simulink library "common_lib"  (R2021b)
settings: Solver=ode45  StartTime=0.0  StopTime=10.0  RelTol=1e-3
undefined symbols (not defined in the file or in its folder): ACCEL_PRE_MULT, C_C1GearNumbers, C_C1GearRatios, C_Calibration, C_DitherWaveform, C_GearOffset, C_GearRatioIn, C_GearRatioInverseOut, C_GearRatioOut, CLUTCH_INNER_LOOP_UPDATE_RATE, CONSTANT, DEGRADED_MODE_SIZE, Dem_EventStatusType, DiscIntNeverNeededParam, F_FAULT_ENUM, F_NOFAULT, F_OUTOFRANGE, F_RATELIMIT, FALSE, FMI14_SPECIAL_INSTRUCTIONS, FMI20_DATA_DRIFTED_HIGH, FMI21_DATA_DRIFTED_LOW, FMI29_RESERVED_FOR_SAE_ASSIGNMENT, FMI30_RESERVED_FOR_SAE_ASSIGNMENT, FMI31_CONDITION_EXISTS, FMI32_NO_FAULT, IC, k_accel, k_mean, LVDCU_OORH_FaultCntThd_C, MAX_UINT32, MEAN_PRE_MULT, NTriggers, QLTY_SIGNAL_FAILED, QLTY_SIGNAL_FULLY_FUNCTION, QLTY_SIGNAL_SUBSTITUTED_BY_1ST_CHOICE, QLTY_SIGNAL_SUBSTITUTED_BY_2ND_CHOICE, QLTY_SIGNAL_SUBSTITUTED_BY_3RD_CHOICE, QLTY_SIGNAL_SUBSTITUTED_BY_4TH_CHOICE, SAMPLE_TIME_100_mSec, SAMPLE_TIME_100_uSec, simin, T_TestPoint, TF_FALSE, TF_TRUE, TimeStep, TRUE, WORKSPACE_UPDATE_RATE, ZERO, Zero
libraries: $bdroot x120, simulink x27, simulink_extras x4, MBD_EPS_Local_Blockset x4
(part 10 of 10)

== stateflow chart common_lib/Diagnostics/DiagcFltStSpaceHoldCnt/diagcounter_hold ==
  state Init
    en: diagFaultCnt = int16(0);
    diagFaultStatus = PASSED;
    Init -> (junction 169) [order 1]
    (junction 169) -> (junction 170) [order 1] : [~diagStartUpComp || diagReset]
        | {diagFaultCnt = int16(0);}
    (junction 169) -> (junction 171) [order 2]
    (junction 170) -> (junction 180)
    (junction 171) -> (junction 172) [order 1] : [~diagFaultActive]
    (junction 171) -> (junction 173) [order 2]
    (junction 172) -> (junction 179) : {diagFaultCnt = diagFaultCnt;}
    (junction 173) -> (junction 174) [order 1] : [diagFaultActive]
    (junction 174) -> (junction 175) [order 1] : [diagFaultCnt>=diagFaultCntThresh]
        | {diagFaultStatus = FAILED}
    (junction 173) -> (junction 176) [order 2]
    (junction 174) -> (junction 177) [order 2] : {diagFaultCnt = diagFaultCnt + diagUpCnt;}
    (junction 175) -> (junction 178)
    (junction 177) -> (junction 176)
    (junction 178) -> (junction 177)
    (junction 179) -> (junction 178)
    (junction 180) -> (junction 179)
    (junction 176) -> (junction 181)
  state Fault
    en:
    diagFaultStatus = FAILED ;
    Fault -> (junction 200) [order 1]
    (junction 200) -> (junction 201) [order 1] : [(diagFaultCnt<diagFaultCntThresh) && diagFaultActive]
        | {diagFaultCnt = diagFaultCnt + diagUpCnt;}
    (junction 200) -> (junction 202) [order 2]
    (junction 201) -> (junction 203)
    (junction 203) -> (junction 202)
    (junction 202) -> (junction 204)
  state Pass
    en: diagFaultCnt = int16(0);
    diagFaultStatus = PASSED;
    Pass -> (junction 212) [order 1]
    (junction 212) -> (junction 213) [order 1] : [(diagFaultCnt>int16(0)) && ~diagFaultActive]
        | {diagFaultCnt = diagFaultCnt;}
    (junction 212) -> (junction 215) [order 2]
    (junction 213) -> (junction 221)
    (junction 215) -> (junction 216) [order 1] : [diagFaultActive]
    (junction 216) -> (junction 217) [order 1] : [diagFaultCnt>=diagFaultCntThresh]
        | {diagFaultStatus = FAILED;}
    (junction 215) -> (junction 218) [order 2]
    (junction 216) -> (junction 219) [order 2] : {diagFaultCnt = diagFaultCnt + diagUpCnt;}
    (junction 217) -> (junction 220)
    (junction 219) -> (junction 218)
    (junction 220) -> (junction 219)
    (junction 221) -> (junction 220)
    (junction 218) -> (junction 223)
  (default) -> Init : {diagFaultStatus = PASSED
      | diagFaultCnt = int16(0)}
  Init -> Fault [order 1] : [diagFaultCnt>=diagFaultCntThresh &&...
      | diagStartUpComp &&...
      | ~diagReset]
  Fault -> Init [order 2] : [~diagStartUpComp ||...
      | diagReset]
  Fault -> Pass [order 1] : [diagReset]
  Pass -> Fault [order 1] : [diagFaultCnt>=diagFaultCntThresh]
  Init -> Pass [order 2] : [diagFaultCnt==0&&...
      | diagStartUpComp...
      |  &&~diagReset]
  Pass -> Init [order 2] : [~diagStartUpComp ||...
      | diagReset]
  data: diagFaultActive input; diagStartUpComp input; diagUpCnt input; diagFaultCntThresh input; diagReset input; diagFaultStatus output; diagFaultCnt output; FAILED constant boolean =1; PASSED constant boolean =0

== stateflow chart common_lib/Bit/uint8 Bit Pack ==
  settings: stateMachineType=MEALY_MACHINE
  (default) -> (junction 10) : {Byte=0;}
  (junction 10) -> (junction 13) [order 1] : [Bit_0]{Byte=Byte | 1;}
  (junction 10) -> (junction 13) [order 2]
  (junction 13) -> (junction 20) [order 1] : [Bit_1]{Byte=Byte | 2;}
  (junction 13) -> (junction 20) [order 2]
  (junction 20) -> (junction 26) [order 1] : [Bit_2]{Byte=Byte | 4;}
  (junction 20) -> (junction 26) [order 2]
  (junction 26) -> (junction 31) [order 1] : [Bit_3]{Byte=Byte | 8;}
  (junction 26) -> (junction 31) [order 2]
  (junction 31) -> (junction 36) [order 1] : [Bit_4]{Byte=Byte | 16;}
  (junction 31) -> (junction 36) [order 2]
  (junction 36) -> (junction 41) [order 1] : [Bit_5]{Byte=Byte | 32;}
  (junction 36) -> (junction 41) [order 2]
  (junction 41) -> (junction 46) [order 1] : [Bit_6]{Byte=Byte | 64;}
  (junction 41) -> (junction 46) [order 2]
  (junction 46) -> (junction 51) [order 1] : [Bit_7]{Byte=Byte | 128;}
  (junction 46) -> (junction 51) [order 2]
  data: Bit_0 input boolean size=1; Bit_1 input boolean size=1; Bit_2 input boolean size=1; Bit_3 input boolean size=1; Bit_4 input boolean size=1; Bit_5 input boolean size=1; Bit_6 input boolean size=1; Bit_7 input boolean size=1; Byte output uint8 size=1

== stateflow chart common_lib/Bit/uint8 Bit Unpack ==
  settings: stateMachineType=MEALY_MACHINE
  (default) -> (junction 17) : {Bit_0 = Byte & 1;
      |  Bit_1 = Byte & 2;
      |  Bit_2 = Byte & 4;
      |  Bit_3 = Byte & 8;
      |  Bit_4 = Byte & 16;
      |  Bit_5 = Byte & 32;
      |  Bit_6 = Byte & 64;
      |  Bit_7 = Byte & 128;}
  data: Byte input uint8 size=1; Bit_0 output boolean size=1; Bit_1 output boolean size=1; Bit_2 output boolean size=1; Bit_3 output boolean size=1; Bit_4 output boolean size=1; Bit_5 output boolean size=1; Bit_6 output boolean size=1; Bit_7 output boolean size=1

== stateflow chart common_lib/Bit/uint16 Bit Pack ==
  settings: stateMachineType=MEALY_MACHINE
  (default) -> (junction 10) : {Byte=0;}
  (junction 10) -> (junction 13) [order 1] : [Bit_0]{Byte=Byte | 1;}
  (junction 10) -> (junction 13) [order 2]
  (junction 13) -> (junction 20) [order 1] : [Bit_1]{Byte=Byte | 2;}
  (junction 13) -> (junction 20) [order 2]
  (junction 20) -> (junction 26) [order 1] : [Bit_2]{Byte=Byte | 4;}
  (junction 20) -> (junction 26) [order 2]
  (junction 26) -> (junction 31) [order 1] : [Bit_3]{Byte=Byte | 8;}
  (junction 26) -> (junction 31) [order 2]
  (junction 31) -> (junction 36) [order 1] : [Bit_4]{Byte=Byte | 16;}
  (junction 31) -> (junction 36) [order 2]
  (junction 36) -> (junction 41) [order 1] : [Bit_5]{Byte=Byte | 32;}
  (junction 36) -> (junction 41) [order 2]
  (junction 41) -> (junction 46) [order 1] : [Bit_6]{Byte=Byte | 64;}
  (junction 41) -> (junction 46) [order 2]
  (junction 46) -> (junction 65) [order 1] : [Bit_7]{Byte=Byte | 128;}
  (junction 46) -> (junction 65) [order 2]
  (junction 65) -> (junction 66) [order 1] : [Bit_8]{Byte=Byte | 256;}
  (junction 65) -> (junction 66) [order 2]
  (junction 66) -> (junction 69) [order 1] : [Bit_9]{Byte=Byte | 512;}
  (junction 66) -> (junction 69) [order 2]
  (junction 69) -> (junction 72) [order 1] : [Bit_10]{Byte=Byte | 1024;}
  (junction 69) -> (junction 72) [order 2]
  (junction 72) -> (junction 73) [order 1] : [Bit_11]{Byte=Byte | 2048;}
  (junction 72) -> (junction 73) [order 2]
  (junction 73) -> (junction 68) [order 1] : [Bit_12]{Byte=Byte | 4096;}
  (junction 73) -> (junction 68) [order 2]
  (junction 68) -> (junction 71) [order 1] : [Bit_13]{Byte=Byte | 8192;}
  (junction 68) -> (junction 71) [order 2]
  (junction 71) -> (junction 70) [order 1] : [Bit_14]{Byte=Byte | 16384;}
  (junction 71) -> (junction 70) [order 2]
  (junction 70) -> (junction 67) [order 1] : [Bit_15]{Byte=Byte | 32768;}
  (junction 70) -> (junction 67) [order 2]
  data: Bit_0 input boolean size=1; Bit_1 input boolean size=1; Bit_2 input boolean size=1; Bit_3 input boolean size=1; Bit_4 input boolean size=1; Bit_5 input boolean size=1; Bit_6 input boolean size=1; Bit_7 input boolean size=1; Byte output uint16 size=1; Bit_8 input boolean size=1; Bit_9 input boolean size=1; Bit_10 input boolean size=1; Bit_11 input boolean size=1; Bit_12 input boolean size=1; Bit_13 input boolean size=1; Bit_14 input boolean size=1; Bit_15 input boolean size=1

== stateflow chart common_lib/Bit/uint16 Bit Unpack ==
  settings: stateMachineType=MEALY_MACHINE
  (default) -> (junction 17) : {Bit_0 = Byte & 1;
      |  Bit_1 = Byte & 2;
      |  Bit_2 = Byte & 4;
      |  Bit_3 = Byte & 8;
      |  Bit_4 = Byte & 16;
      |  Bit_5 = Byte & 32;
      |  Bit_6 = Byte & 64;
      |  Bit_7 = Byte & 128;
      |  Bit_8 = Byte & 256;
      |  Bit_9 = Byte & 512;
      |  Bit_10 = Byte & 1024;
      |  Bit_11 = Byte & 2048;
      |  Bit_12 = Byte & 4096;
      |  Bit_13 = Byte & 8192;
      |  Bit_14 = Byte & 16384;
      |  Bit_15 = Byte & 32768;}
  data: Byte input uint16 size=1; Bit_0 output boolean size=1; Bit_1 output boolean size=1; Bit_2 output boolean size=1; Bit_3 output boolean size=1; Bit_4 output boolean size=1; Bit_5 output boolean size=1; Bit_6 output boolean size=1; Bit_7 output boolean size=1; Bit_8 output boolean size=1; Bit_9 output boolean size=1; Bit_10 output boolean size=1; Bit_11 output boolean size=1; Bit_12 output boolean size=1; Bit_13 output boolean size=1; Bit_14 output boolean size=1; Bit_15 output boolean size=1

== stateflow chart common_lib/Diagnostics/Calibration Enabled Debounce Boolean Input/DiagFaultCounter/DiagFaulCounter ==
  state FaultDebounceDisabled
    en: diagFaultStatus = PASSED;
    diagFaultCnt = int16(0);
    FaultDebounceDisabled -> (junction 32) [order 1]
    (junction 32) -> (junction 29) [order 1] : [~diagStartUpComp || diagReset || ~diagEnable]
        | {diagFaultStatus = PASSED;}
    (junction 32) -> (junction 23) [order 2]
    (junction 29) -> (junction 27)
    (junction 23) -> (junction 24) [order 1] : [~diagFaultActive]
        | {diagFaultStatus = PASSED;}
    (junction 23) -> (junction 26) [order 2]
    (junction 24) -> (junction 282)
    (junction 26) -> (junction 281) [order 1] : [diagFaultActive]
        | {diagFaultStatus = FAILED;}
    (junction 26) -> (junction 51) [order 2]
    (junction 281) -> (junction 283)
    (junction 283) -> (junction 51)
    (junction 282) -> (junction 283)
    (junction 27) -> (junction 282)
    (junction 51) -> (junction 288)
  state FaultDebounceEnabled
    en: diagFaultStatus = PASSED;
    diagFaultCnt = int16(0);
    state Init
      en: diagFaultCnt = int16(0);
      diagFaultStatus = PASSED;
      Init -> (junction 248) [order 1]
      (junction 248) -> (junction 249) [order 1] : [~diagStartUpComp || diagReset || ~diagEnable]
          | {diagFaultCnt = int16(0);}
      (junction 248) -> (junction 250) [order 2]
      (junction 249) -> (junction 257)
      (junction 253) -> (junction 342) [order 1] : [diagFaultCnt<=diagPassCntThresh]
          | {diagFaultStatus = PASSED;}
      (junction 250) -> (junction 253) [order 1] : [~diagFaultActive]
      (junction 250) -> (junction 252) [order 2]
      (junction 253) -> (junction 255) [order 2] : {diagFaultCnt = diagFaultCnt - diagDnCnt;}
      (junction 342) -> (junction 344)
      (junction 251) -> (junction 310) [order 1] : [diagFaultCnt>=diagFaultCntThresh]
          | {diagFaultStatus = FAILED}
      (junction 252) -> (junction 251) [order 1] : [diagFaultActive]
      (junction 252) -> (junction 254) [order 2]
      (junction 251) -> (junction 256) [order 2] : {diagFaultCnt = diagFaultCnt + diagUpCnt;}
      (junction 310) -> (junction 338)
      (junction 256) -> (junction 254)
      (junction 338) -> (junction 256)
      (junction 255) -> (junction 338)
      (junction 344) -> (junction 255)
      (junction 257) -> (junction 344)
      (junction 254) -> (junction 258)
    state Fault
      en: diagFaultCnt = int16(0);
      diagFaultStatus = FAILED ;
      Fault -> (junction 133) [order 1]
      (junction 133) -> (junction 134) [order 1] : [(diagFaultCnt<int16(0)) && diagFaultActive]
          | {diagFaultCnt = diagFaultCnt + diagUpCnt;}
      (junction 134) -> (junction 152) [order 1] : [diagFaultCnt>int16(0)]
          | {diagFaultCnt = int16(0)}
      (junction 133) -> (junction 135) [order 2]
      (junction 134) -> (junction 139) [order 2]
      (junction 152) -> (junction 155)
      (junction 135) -> (junction 136) [order 1] : [~diagFaultActive && diagHealEn]
      (junction 136) -> (junction 298) [order 1] : [diagFaultCnt<=diagPassCntThresh]
          | {diagFaultStatus = PASSED;}
      (junction 135) -> (junction 137) [order 2]
      (junction 136) -> (junction 138) [order 2] : {diagFaultCnt = diagFaultCnt - diagDnCnt;}
      (junction 298) -> (junction 300)
      (junction 138) -> (junction 137)
      (junction 300) -> (junction 138)
      (junction 139) -> (junction 300)
      (junction 155) -> (junction 139)
      (junction 137) -> (junction 140)
    state Pass
      en: diagFaultCnt = int16(0);
      diagFaultStatus = PASSED;
      Pass -> (junction 159) [order 1]
      (junction 159) -> (junction 160) [order 1] : [(diagFaultCnt>int16(0)) && ~diagFaultActive]
          | {diagFaultCnt = diagFaultCnt - diagDnCnt;}
      (junction 160) -> (junction 161) [order 1] : [diagFaultCnt<int16(0)]
          | {diagFaultCnt = int16(0)}
      (junction 159) -> (junction 162) [order 2]
      (junction 160) -> (junction 166) [order 2]
      (junction 161) -> (junction 167)
      (junction 162) -> (junction 163) [order 1] : [diagFaultActive]
      (junction 163) -> (junction 305) [order 1] : [diagFaultCnt>=diagFaultCntThresh]
          | {diagFaultStatus = FAILED;}
      (junction 162) -> (junction 164) [order 2]
      (junction 163) -> (junction 165) [order 2] : {diagFaultCnt = diagFaultCnt + diagUpCnt;}
      (junction 305) -> (junction 304)
      (junction 165) -> (junction 164)
      (junction 304) -> (junction 165)
      (junction 166) -> (junction 304)
      (junction 167) -> (junction 166)
      (junction 164) -> (junction 168)
    (default) -> Init
    Init -> Fault [order 1] : [diagFaultCnt>=diagFaultCntThresh &&...
        | diagStartUpComp &&...
        | ~diagReset && diagEnable]
    Fault -> Init [order 2] : [~diagStartUpComp ||...
        | diagReset || ~diagEnable]
    Fault -> Pass [order 1] : [diagFaultCnt<=diagPassCntThresh && diagHealEn]
    Pass -> Fault [order 1] : [diagFaultCnt>=diagFaultCntThresh]
    Init -> Pass [order 2] : [diagFaultCnt<=diagPassCntThresh &&...
        | diagStartUpComp &&...
        | ~diagReset && diagEnable]
    Pass -> Init [order 2] : [~diagStartUpComp ||...
        | diagReset || ~diagEnable]
  (default) -> (junction 58)
  (junction 58) -> (junction 279) [order 2]
  (junction 58) -> FaultDebounceEnabled [order 1] : [diagDbncEnab]
  (junction 279) -> FaultDebounceDisabled
  FaultDebounceEnabled -> FaultDebounceDisabled : [~diagDbncEnab]
  FaultDebounceDisabled -> FaultDebounceEnabled [order 1] : [diagDbncEnab]
  data: diagFaultActive input boolean size=1; diagStartUpComp input boolean size=1; diagReset input boolean size=1; diagEnable input boolean size=1; diagDbncEnab input boolean size=1; diagFaultCntThresh input int16 size=1; diagPassCntThresh input int16 size=1; diagUpCnt input int16 size=1; diagDnCnt input int16 size=1; diagFaultStatus output size=1; diagHealEn input boolean size=1; PASSED constant boolean =0; FAILED constant boolean =1; diagFaultCnt output int16 size=1

== stateflow chart common_lib/Diagnostics/DiagFaultCounter/DiagFaulCounter ==
  state FaultDebounceDisabled
    en: diagFaultStatus = Dem_EventStatusType.DEM_EVENT_STATUS_INIT;
    diagFaultCnt = int16(0);
    FaultDebounceDisabled -> (junction 32) [order 1]
    (junction 32) -> (junction 29) [order 1] : [~diagStartUpComp || diagReset || ~diagEnable]
        | {diagFaultStatus = Dem_EventStatusType.DEM_EVENT_STATUS_INIT;}
    (junction 32) -> (junction 23) [order 2]
    (junction 29) -> (junction 27)
    (junction 23) -> (junction 24) [order 1] : [~diagFaultActive]
        | {diagFaultStatus = Dem_EventStatusType.DEM_EVENT_STATUS_PREPASSED;}
    (junction 23) -> (junction 26) [order 2]
    (junction 24) -> (junction 282)
    (junction 26) -> (junction 281) [order 1] : [diagFaultActive]
        | {diagFaultStatus = Dem_EventStatusType.DEM_EVENT_STATUS_PREFAILED;}
    (junction 26) -> (junction 51) [order 2]
    (junction 281) -> (junction 283)
    (junction 283) -> (junction 51)
    (junction 282) -> (junction 283)
    (junction 27) -> (junction 282)
    (junction 51) -> (junction 288)
  state FaultDebounceEnabled
    en: diagFaultStatus = Dem_EventStatusType.DEM_EVENT_STATUS_INIT;
    diagFaultCnt = int16(0);
    state Init
      en: diagFaultCnt = int16(0);
      diagFaultStatus = Dem_EventStatusType.DEM_EVENT_STATUS_INIT;
      Init -> (junction 248) [order 1]
      (junction 248) -> (junction 249) [order 1] : [~diagStartUpComp || diagReset || ~diagEnable]
          | {diagFaultCnt = int16(0);}
      (junction 248) -> (junction 250) [order 2]
      (junction 249) -> (junction 257)
      (junction 250) -> (junction 253) [order 1] : [~diagFaultActive]
      (junction 253) -> (junction 342) [order 1] : [diagFaultCnt<=diagPassCntThresh]
          | {diagFaultStatus = Dem_EventStatusType.DEM_EVENT_STATUS_PASSED;}
      (junction 250) -> (junction 252) [order 2]
      (junction 253) -> (junction 255) [order 2] : {diagFaultCnt = diagFaultCnt - diagDnCnt;}
      (junction 342) -> (junction 344)
      (junction 252) -> (junction 251) [order 1] : [diagFaultActive]
      (junction 251) -> (junction 310) [order 1] : [diagFaultCnt>=diagFaultCntThresh]
          | {diagFaultStatus = Dem_EventStatusType.DEM_EVENT_STATUS_FAILED;}
      (junction 252) -> (junction 254) [order 2]
      (junction 251) -> (junction 256) [order 2] : {diagFaultCnt = diagFaultCnt + diagUpCnt;}
      (junction 310) -> (junction 338)
      (junction 256) -> (junction 254)
      (junction 338) -> (junction 256)
      (junction 255) -> (junction 338)
      (junction 344) -> (junction 255)
      (junction 257) -> (junction 344)
      (junction 254) -> (junction 258)
    state Fault
      en: diagFaultCnt = int16(0);
      diagFaultStatus = Dem_EventStatusType.DEM_EVENT_STATUS_FAILED;
      Fault -> (junction 133) [order 1]
      (junction 133) -> (junction 134) [order 1] : [(diagFaultCnt<int16(0)) && diagFaultActive]
          | {diagFaultCnt = diagFaultCnt + diagUpCnt;}
      (junction 134) -> (junction 152) [order 1] : [diagFaultCnt>int16(0)]
          | {diagFaultCnt = int16(0)}
      (junction 133) -> (junction 135) [order 2]
      (junction 134) -> (junction 139) [order 2]
      (junction 152) -> (junction 155)
      (junction 136) -> (junction 298) [order 1] : [diagFaultCnt<=diagPassCntThresh]
          | {diagFaultStatus = Dem_EventStatusType.DEM_EVENT_STATUS_PASSED;}
      (junction 135) -> (junction 136) [order 1] : [~diagFaultActive && diagHealEn]
      (junction 135) -> (junction 137) [order 2]
      (junction 298) -> (junction 300)
      (junction 136) -> (junction 138) [order 2] : {diagFaultCnt = diagFaultCnt - diagDnCnt;}
      (junction 138) -> (junction 137)
      (junction 300) -> (junction 138)
      (junction 139) -> (junction 300)
      (junction 155) -> (junction 139)
      (junction 137) -> (junction 140)
    state Pass
      en: diagFaultCnt = int16(0);
      diagFaultStatus = Dem_EventStatusType.DEM_EVENT_STATUS_PASSED;
      Pass -> (junction 159) [order 1]
      (junction 159) -> (junction 160) [order 1] : [(diagFaultCnt>int16(0)) && ~diagFaultActive]
          | {diagFaultCnt = diagFaultCnt - diagDnCnt;}
      (junction 160) -> (junction 161) [order 1] : [diagFaultCnt<int16(0)]
          | {diagFaultCnt = int16(0)}
      (junction 159) -> (junction 162) [order 2]
      (junction 160) -> (junction 166) [order 2]
      (junction 161) -> (junction 167)
      (junction 163) -> (junction 305) [order 1] : [diagFaultCnt>=diagFaultCntThresh]
          | {diagFaultStatus = Dem_EventStatusType.DEM_EVENT_STATUS_FAILED;}
      (junction 162) -> (junction 163) [order 1] : [diagFaultActive]
      (junction 162) -> (junction 164) [order 2]
      (junction 305) -> (junction 304)
      (junction 163) -> (junction 165) [order 2] : {diagFaultCnt = diagFaultCnt + diagUpCnt;}
      (junction 165) -> (junction 164)
      (junction 304) -> (junction 165)
      (junction 166) -> (junction 304)
      (junction 167) -> (junction 166)
      (junction 164) -> (junction 168)
    (default) -> Init
    Init -> Fault [order 1] : [diagFaultCnt>=diagFaultCntThresh &&...
        | diagStartUpComp &&...
        | ~diagReset && diagEnable]
    Fault -> Init [order 2] : [~diagStartUpComp ||...
        | diagReset || ~diagEnable]
    Fault -> Pass [order 1] : [diagFaultCnt<=diagPassCntThresh && diagHealEn]
    Pass -> Fault [order 1] : [diagFaultCnt>=diagFaultCntThresh]
    Init -> Pass [order 2] : [diagFaultCnt<=diagPassCntThresh &&...
        | diagStartUpComp &&...
        | ~diagReset && diagEnable]
    Pass -> Init [order 2] : [~diagStartUpComp ||...
        | diagReset || ~diagEnable]
  (default) -> (junction 58)
  (junction 58) -> (junction 279) [order 2]
  (junction 58) -> FaultDebounceEnabled [order 1] : [diagDbncEnab]
  (junction 279) -> FaultDebounceDisabled
  FaultDebounceEnabled -> FaultDebounceDisabled : [~diagDbncEnab]
  FaultDebounceDisabled -> FaultDebounceEnabled [order 1] : [diagDbncEnab]
  data: diagFaultActive input boolean size=1; diagStartUpComp input boolean size=1; diagReset input boolean size=1; diagEnable input boolean size=1; diagDbncEnab input boolean size=1; diagFaultCntThresh input int16 size=1; diagPassCntThresh input int16 size=1; diagUpCnt input int16 size=1; diagDnCnt input int16 size=1; diagFaultStatus output size=1; diagHealEn input boolean size=1; diagFaultCnt local int16 size=1

== stateflow chart common_lib/Diagnostics/DiagcFltStSpaceRstCnt/Chart ==
  state FaultDebounceEnabled
    en: diagFaultCnt = int16(0);
    state Init
      en: diagFaultCnt =int16(0);
      (junction 36) -> (junction 37) [order 1] : [~diagStartUpComp || diagReset]
          | {diagFaultCnt =int16(0);}
      Init -> (junction 36) [order 1]
      (junction 36) -> (junction 38) [order 2]
      (junction 37) -> (junction 49)
      (junction 38) -> (junction 39) [order 1] : [~diagFaultActive]
      (junction 38) -> (junction 41) [order 2]
      (junction 39) -> (junction 47) : {diagFaultCnt =int16(0);}
      (junction 41) -> (junction 42) [order 1] : [diagFaultActive]
      (junction 42) -> (junction 43) [order 1] : [diagFaultCnt>=diagFaultCntThresh]
          | {diagFaultStatus = FAILED}
      (junction 41) -> (junction 44) [order 2]
      (junction 42) -> (junction 45) [order 2] : {diagFaultCnt = diagFaultCnt + diagUpCnt;}
      (junction 43) -> (junction 46)
      (junction 45) -> (junction 44)
      (junction 46) -> (junction 45)
      (junction 47) -> (junction 46)
      (junction 49) -> (junction 47)
      (junction 44) -> (junction 50)
    state Fault
      en:
      diagFaultStatus = FAILED ;
      Fault -> (junction 72) [order 1]
      (junction 72) -> (junction 73) [order 1] : [(diagFaultCnt<diagFaultCntThresh) && diagFaultActive]
          | {diagFaultCnt = diagFaultCnt + diagUpCnt;}
      (junction 72) -> (junction 78) [order 2]
      (junction 73) -> (junction 81)
      (junction 81) -> (junction 78)
      (junction 78) -> (junction 83)
    state Pass
      en: diagFaultCnt = int16(0);
      diagFaultStatus = PASSED;
      Pass -> (junction 101) [order 1]
      (junction 101) -> (junction 102) [order 1] : [(diagFaultCnt>int16(0)) && ~diagFaultActive]
          | {diagFaultCnt =int16(0);}
      (junction 101) -> (junction 104) [order 2]
      (junction 102) -> (junction 110)
      (junction 104) -> (junction 105) [order 1] : [diagFaultActive]
      (junction 105) -> (junction 106) [order 1] : [diagFaultCnt>=diagFaultCntThresh]
          | {diagFaultStatus = FAILED;}
      (junction 104) -> (junction 107) [order 2]
      (junction 105) -> (junction 108) [order 2] : {diagFaultCnt = diagFaultCnt + diagUpCnt;}
      (junction 106) -> (junction 109)
      (junction 108) -> (junction 107)
      (junction 109) -> (junction 108)
      (junction 110) -> (junction 109)
      (junction 107) -> (junction 112)
    (default) -> Init
    Init -> Fault [order 1] : [diagFaultCnt>=diagFaultCntThresh &&...
        | diagStartUpComp &&...
        | ~diagReset]
    Fault -> Init [order 2] : [~diagStartUpComp ||...
        | diagReset]
    Fault -> Pass [order 1] : [diagReset]
    Pass -> Fault [order 1] : [diagFaultCnt>=diagFaultCntThresh]
    Init -> Pass [order 2] : [diagFaultCnt==0&&...
        | diagStartUpComp...
        |  &&~diagReset]
    Pass -> Init [order 2] : [~diagStartUpComp ||...
        | diagReset]
  data: diagFaultActive input; diagStartUpComp input; diagUpCnt input; diagFaultCntThresh input; diagReset input; diagFaultStatus output; FAILED constant boolean =1; PASSED constant boolean =0; diagFaultCnt output

== stateflow chart common_lib/Diagnostics/DTNA_Diag/S_Diag/DiagFaultCounter/DiagFaulCounter ==
  state FaultDebounceDisabled
    en: diagFaultStatus = PASSED;
    diagFaultCnt = int16(0);
    FaultDebounceDisabled -> (junction 32) [order 1]
    (junction 32) -> (junction 29) [order 1] : [~diagStartUpComp || diagReset || ~diagEnable]
        | {diagFaultStatus = PASSED;}
    (junction 32) -> (junction 23) [order 2]
    (junction 29) -> (junction 27)
    (junction 23) -> (junction 24) [order 1] : [~diagFaultActive]
        | {diagFaultStatus = PASSED;}
    (junction 23) -> (junction 26) [order 2]
    (junction 24) -> (junction 282)
    (junction 26) -> (junction 281) [order 1] : [diagFaultActive]
        | {diagFaultStatus = FAILED;}
    (junction 26) -> (junction 51) [order 2]
    (junction 281) -> (junction 283)
    (junction 283) -> (junction 51)
    (junction 282) -> (junction 283)
    (junction 27) -> (junction 282)
    (junction 51) -> (junction 288)
  state FaultDebounceEnabled
    en: diagFaultStatus = PASSED;
    diagFaultCnt = int16(0);
    state Init
      en: diagFaultCnt = int16(0);
      diagFaultStatus = PASSED;
      Init -> (junction 248) [order 1]
      (junction 248) -> (junction 249) [order 1] : [~diagStartUpComp || diagReset || ~diagEnable]
          | {diagFaultCnt = int16(0);}
      (junction 248) -> (junction 250) [order 2]
      (junction 249) -> (junction 257)
      (junction 253) -> (junction 342) [order 1] : [diagFaultCnt<=diagPassCntThresh]
          | {diagFaultStatus = PASSED;}
      (junction 250) -> (junction 253) [order 1] : [~diagFaultActive]
      (junction 250) -> (junction 252) [order 2]
      (junction 253) -> (junction 255) [order 2] : {diagFaultCnt = diagFaultCnt - diagDnCnt;}
      (junction 342) -> (junction 344)
      (junction 251) -> (junction 310) [order 1] : [diagFaultCnt>=diagFaultCntThresh]
          | {diagFaultStatus = FAILED}
      (junction 252) -> (junction 251) [order 1] : [diagFaultActive]
      (junction 252) -> (junction 254) [order 2]
      (junction 251) -> (junction 256) [order 2] : {diagFaultCnt = diagFaultCnt + diagUpCnt;}
      (junction 310) -> (junction 338)
      (junction 256) -> (junction 254)
      (junction 338) -> (junction 256)
      (junction 255) -> (junction 338)
      (junction 344) -> (junction 255)
      (junction 257) -> (junction 344)
      (junction 254) -> (junction 258)
    state Fault
      en: diagFaultCnt = int16(0);
      diagFaultStatus = FAILED ;
      Fault -> (junction 133) [order 1]
      (junction 133) -> (junction 134) [order 1] : [(diagFaultCnt<int16(0)) && diagFaultActive]
          | {diagFaultCnt = diagFaultCnt + diagUpCnt;}
      (junction 134) -> (junction 152) [order 1] : [diagFaultCnt>int16(0)]
          | {diagFaultCnt = int16(0)}
      (junction 133) -> (junction 135) [order 2]
      (junction 134) -> (junction 139) [order 2]
      (junction 152) -> (junction 155)
      (junction 135) -> (junction 136) [order 1] : [~diagFaultActive && diagHealEn]
      (junction 136) -> (junction 298) [order 1] : [diagFaultCnt<=diagPassCntThresh]
          | {diagFaultStatus = PASSED;}
      (junction 135) -> (junction 137) [order 2]
      (junction 136) -> (junction 138) [order 2] : {diagFaultCnt = diagFaultCnt - diagDnCnt;}
      (junction 298) -> (junction 300)
      (junction 138) -> (junction 137)
      (junction 300) -> (junction 138)
      (junction 139) -> (junction 300)
      (junction 155) -> (junction 139)
      (junction 137) -> (junction 140)
    state Pass
      en: diagFaultCnt = int16(0);
      diagFaultStatus = PASSED;
      Pass -> (junction 159) [order 1]
      (junction 159) -> (junction 160) [order 1] : [(diagFaultCnt>int16(0)) && ~diagFaultActive]
          | {diagFaultCnt = diagFaultCnt - diagDnCnt;}
      (junction 160) -> (junction 161) [order 1] : [diagFaultCnt<int16(0)]
          | {diagFaultCnt = int16(0)}
      (junction 159) -> (junction 162) [order 2]
      (junction 160) -> (junction 166) [order 2]
      (junction 161) -> (junction 167)
      (junction 162) -> (junction 163) [order 1] : [diagFaultActive]
      (junction 163) -> (junction 305) [order 1] : [diagFaultCnt>=diagFaultCntThresh]
          | {diagFaultStatus = FAILED;}
      (junction 162) -> (junction 164) [order 2]
      (junction 163) -> (junction 165) [order 2] : {diagFaultCnt = diagFaultCnt + diagUpCnt;}
      (junction 305) -> (junction 304)
      (junction 165) -> (junction 164)
      (junction 304) -> (junction 165)
      (junction 166) -> (junction 304)
      (junction 167) -> (junction 166)
      (junction 164) -> (junction 168)
    (default) -> Init
    Init -> Fault [order 1] : [diagFaultCnt>=diagFaultCntThresh &&...
        | diagStartUpComp &&...
        | ~diagReset && diagEnable]
    Fault -> Init [order 2] : [~diagStartUpComp ||...
        | diagReset || ~diagEnable]
    Fault -> Pass [order 1] : [diagFaultCnt<=diagPassCntThresh && diagHealEn]
    Pass -> Fault [order 1] : [diagFaultCnt>=diagFaultCntThresh]
    Init -> Pass [order 2] : [diagFaultCnt<=diagPassCntThresh &&...
        | diagStartUpComp &&...
        | ~diagReset && diagEnable]
    Pass -> Init [order 2] : [~diagStartUpComp ||...
        | diagReset || ~diagEnable]
  (default) -> (junction 58)
  (junction 58) -> (junction 279) [order 2]
  (junction 58) -> FaultDebounceEnabled [order 1] : [diagDbncEnab]
  (junction 279) -> FaultDebounceDisabled
  FaultDebounceEnabled -> FaultDebounceDisabled : [~diagDbncEnab]
  FaultDebounceDisabled -> FaultDebounceEnabled [order 1] : [diagDbncEnab]
  data: diagFaultActive input boolean size=1; diagStartUpComp input boolean size=1; diagReset input boolean size=1; diagEnable input boolean size=1; diagDbncEnab input boolean size=1; diagFaultCntThresh input int16 size=1; diagPassCntThresh input int16 size=1; diagUpCnt input int16 size=1; diagDnCnt input int16 size=1; diagFaultStatus output size=1; diagHealEn input boolean size=1; PASSED constant boolean =0; FAILED constant boolean =1; diagFaultCnt output int16 size=1
